simulink model "Lab_Second_Order_Open_Closed_Loop_system"  (R2024b)
settings: Solver=VariableStepAuto  StartTime=0.0  StopTime=10.0  RelTol=1e-3
libraries: simulink x1
settings Model: Creator=Ahmad  LastModifiedBy=Ahmad

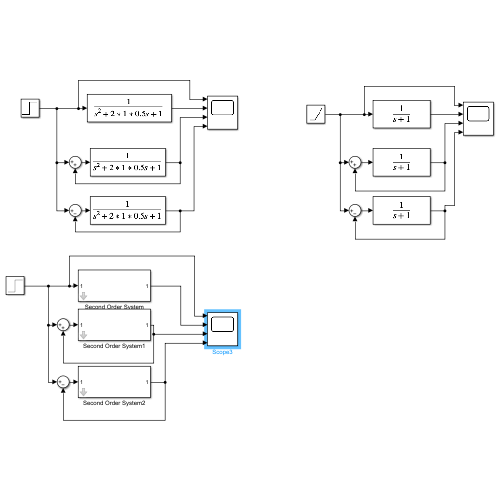
[thumbnail: Simulink's stored preview of the top-level diagram]
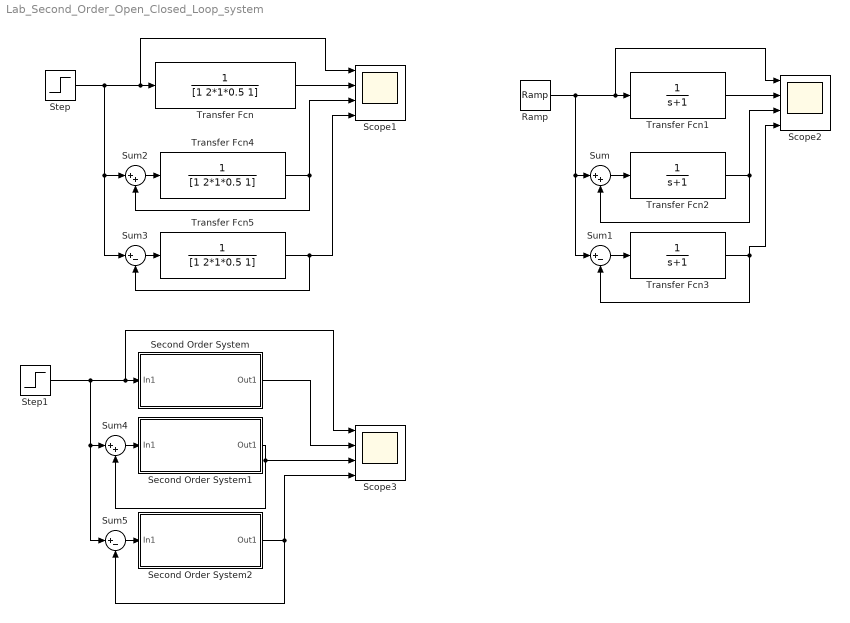
== system Lab_Second_Order_Open_Closed_Loop_system ==
  Ramp : simulink/Sources/Ramp  slope=1  start=0  InitialOutput=0
  Scope1 : Scope  NumInputPorts=4
  Scope2 : Scope  NumInputPorts=4
  Scope3 : Scope  NumInputPorts=4
  Second Order System : Subsystem  mask{Damp_ratio=1, Wn=1}
      mask prompts: Damp_ratio "Damping Ratio"; Wn "Natural Frequency"
  Second Order System1 : Subsystem  mask{Damp_ratio=1, Wn=1}
      mask prompts: Damp_ratio "Damping Ratio"; Wn "Natural Frequency"
  Second Order System2 : Subsystem  mask{Damp_ratio=1, Wn=1}
      mask prompts: Damp_ratio "Damping Ratio"; Wn "Natural Frequency"
  Step : Step  SampleTime=0
  Step1 : Step  SampleTime=0
  Sum : Sum  Inputs=|++
  Sum1 : Sum  Inputs=|+-
  Sum2 : Sum  Inputs=|++
  Sum3 : Sum  Inputs=|+-
  Sum4 : Sum  Inputs=|++
  Sum5 : Sum  Inputs=|+-
  Transfer Fcn : TransferFcn  Denominator=[1 2*1*0.5 1]
  Transfer Fcn1 : TransferFcn  Denominator=[1 1]
  Transfer Fcn2 : TransferFcn  Denominator=[1 1]
  Transfer Fcn3 : TransferFcn  Denominator=[1 1]
  Transfer Fcn4 : TransferFcn  Denominator=[1 2*1*0.5 1]
  Transfer Fcn5 : TransferFcn  Denominator=[1 2*1*0.5 1]
  wires:
  Step/1 -> Scope1/1, Transfer Fcn/1, Sum2/1, Sum3/1
  Ramp/1 -> Sum1/1, Sum/1, Scope2/1, Transfer Fcn1/1
  Sum/1 -> Transfer Fcn2/1
  Transfer Fcn2/1 -> Scope2/3, Sum/2
  Sum1/1 -> Transfer Fcn3/1
  Transfer Fcn3/1 -> Scope2/4, Sum1/2
  Transfer Fcn1/1 -> Scope2/2
  Sum2/1 -> Transfer Fcn4/1
  Transfer Fcn4/1 -> Sum2/2, Scope1/3
  Sum3/1 -> Transfer Fcn5/1
  Transfer Fcn5/1 -> Scope1/4, Sum3/2
  Transfer Fcn/1 -> Scope1/2
  Step1/1 -> Sum5/1, Sum4/1, Scope3/1, Second Order System/1(In1)
  Second Order System/1(Out1) -> Scope3/2
  Sum4/1 -> Second Order System1/1(In1)
  Second Order System1/1(Out1) -> Sum4/2, Scope3/3
  Sum5/1 -> Second Order System2/1(In1)
  Second Order System2/1(Out1) -> Scope3/4, Sum5/2

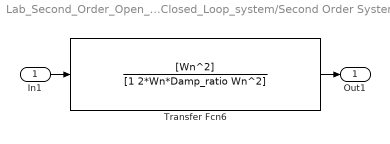
== system Lab_Second_Order_Open_Closed_Loop_system/Second Order System ==
  In1 : Inport
  Transfer Fcn6 : TransferFcn  Numerator=[Wn^2]  Denominator=[1 2*Wn*Damp_ratio Wn^2]
  Out1 : Outport
  wires:
  In1/1 -> Transfer Fcn6/1
  Transfer Fcn6/1 -> Out1/1

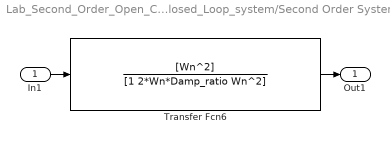
== system Lab_Second_Order_Open_Closed_Loop_system/Second Order System1 ==
  In1 : Inport
  Transfer Fcn6 : TransferFcn  Numerator=[Wn^2]  Denominator=[1 2*Wn*Damp_ratio Wn^2]
  Out1 : Outport
  wires:
  In1/1 -> Transfer Fcn6/1
  Transfer Fcn6/1 -> Out1/1

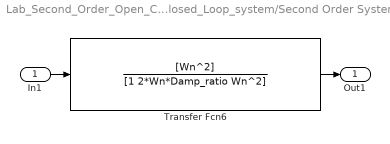
== system Lab_Second_Order_Open_Closed_Loop_system/Second Order System2 ==
  In1 : Inport
  Transfer Fcn6 : TransferFcn  Numerator=[Wn^2]  Denominator=[1 2*Wn*Damp_ratio Wn^2]
  Out1 : Outport
  wires:
  In1/1 -> Transfer Fcn6/1
  Transfer Fcn6/1 -> Out1/1
